simulink model "SHE_4_Angles"  (R2021a)
settings: Solver=daessc  StartTime=0.0  StopTime=.02*20  MaxStep=1e-6  RelTol=1e-3
libraries: spsIGBTDiodeLib x12, spsThreePhaseVIMeasurementLib x3, dsparch4 x2, spsDCVoltageSourceLib x2, spsRMSLib x2, simulink x2, spsVoltageMeasurementLib x2, spsAsynchronousMachineSIUnitsLib x1, spsGroundLib x1, spsThreePhaseSeriesRLCBranchLib x1, spspowerguiLib x1
settings Model: Creator=Ahmed Mohamed  LastModifiedBy=Ahmed Mohamed
settings SolverCC: ZeroCrossAlgorithm=Adaptive
settings DataIOCC: ReturnWorkspaceOutputs=off
settings DebuggingCC: IgnoredZcDiagnostic=none

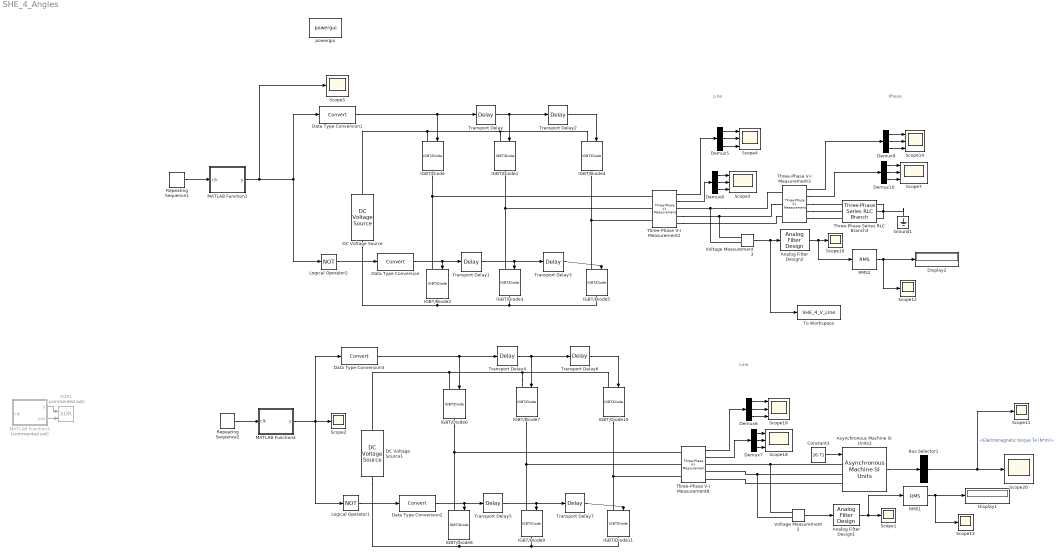
== system SHE_4_Angles ==
  note: Line
  note: Phase
  note: Line
  Analog Filter Design1 : dsparch4/Analog Filter Design  method=Butterworth  filttype=Lowpass  N=8  Wlo=2*pi*500  Whi=80  Rp=2  Rs=40
  Analog Filter Design2 : dsparch4/Analog Filter Design  method=Butterworth  filttype=Lowpass  N=8  Wlo=2*pi*550  Whi=80  Rp=2  Rs=40
  Asynchronous Machine SI Units2 : spsAsynchronousMachineSIUnitsLib/Asynchronous Machine SI Units  RotorType=Squirrel-cage  PresetModel="15:  5.4 HP (4KW)   400 V  50Hz 1430 RPM"  MechanicalLoad=Torque Tm  ShowDetailedParameters=on  ReferenceFrame=Rotor  Units=SI  MeasurementBus=off  NominalParameters=[4000 400 50]  VoltageRatio=1  Stator=[1.405 0.005839]  Rotor=[1.395 0.005839]  Cage1=[0.4155 0.002066]  Cage2=[0.4168 0.0003495]  Lm=0.1722  Mechanical=[0.0131 0.002985 2]  PolePairs=2  InitialConditions=[1 0 0 0 0 0 0 0]  SimulateSaturation=off  Saturation=[14.03593122, 27.81365428, 53.79336849, 72.68890987, 97.98006896, 148.6815601, 215.7428561, 302.9841135, 428.7778367 ; 230, 322, 414, 460, 506, 552, 598, 644, 690]  LoadFlowParameters=1492000  TsPowergui=0  TsBlock=-1  IterativeModel=Trapezoidal non iterative  IterativeDiscreteModel=Trapezoidal non iterative  Pmec=1.492e+006
  Bus Selector1 : BusSelector  OutputSignals=Mechanical.Electromagnetic torque Te (N*m)
  Constant3 : Constant  Value=26.71
  DC Voltage Source : spsDCVoltageSourceLib/DC Voltage Source  Amplitude=558.9759276  Measurements=None
  DC Voltage Source1 : spsDCVoltageSourceLib/DC Voltage Source  Amplitude=558.9759276  Measurements=None
  Data Type Conversion{,1..3} (4 alike) : DataTypeConversion
  Demux{5..10} (6 alike) : Demux  Outputs=3
  Display1 : Display
  Display2 : Display
  Ground1 : spsGroundLib/Ground  LConnTagsString=a
  IGBT/Diode{,1..11} (12 alike) : spsIGBTDiodeLib/IGBT//Diode  Ron=1e-3  Rs=1e5  Cs=inf  Measurements=off
  Logical Operator1 : Logic  Operator=NOT  AllPortsSameDT=off  OutDataTypeStr=boolean
  Logical Operator2 : Logic  Operator=NOT  AllPortsSameDT=off  OutDataTypeStr=boolean
  MATLAB Function1 : MATLAB Function  TreatAsAtomicUnit=on
  MATLAB Function3 : MATLAB Function  Commented=on  TreatAsAtomicUnit=on
  MATLAB Function4 : MATLAB Function  TreatAsAtomicUnit=on
  RMS1 : spsRMSLib/RMS  TrueRMS=off  Freq=50  RMSInit=0  Ts=0
  RMS2 : spsRMSLib/RMS  TrueRMS=off  Freq=50  RMSInit=0  Ts=0
  Repeating Sequence1 : simulink/Sources/Repeating Sequence  rep_seq_t=[0 .02]  rep_seq_y=[0 .02]
  Repeating Sequence2 : simulink/Sources/Repeating Sequence  rep_seq_t=[0 .02]  rep_seq_y=[0 .02]
  Scope{1..2,5,10..13,20} (8 alike) : Scope
  Scope{3..4,7,14,18..19} (6 alike) : Scope  NumInputPorts=3
  Three-Phase Series RLC Branch3 : spsThreePhaseSeriesRLCBranchLib/Three-Phase Series RLC Branch  LConnTagsString=A|B|C  RConnTagsString=A|B|C  BranchType=RL  Resistance=7.5*sqrt(2)  Inductance=7.5*sqrt(2)/314  Capacitance=1e-6  Measurements=None
  Three-Phase V-I Measurement2 : spsThreePhaseVIMeasurementLib/Three-Phase V-I Measurement  VoltageMeasurement=phase-to-phase  SetLabelV=off  LabelV=Vabc  Vpu=off  VpuLL=off  CurrentMeasurement=yes  SetLabelI=off  LabelI=Iabc  Ipu=off  Pbase=100e6  Vbase=500e3  OutputType=Complex  PhasorSimulation=off  PSBequivalent=0
  Three-Phase V-I Measurement3 : spsThreePhaseVIMeasurementLib/Three-Phase V-I Measurement  VoltageMeasurement=phase-to-ground  SetLabelV=off  LabelV=Vabc  Vpu=off  VpuLL=off  CurrentMeasurement=yes  SetLabelI=off  LabelI=Iabc  Ipu=off  Pbase=100e6  Vbase=500e3  OutputType=Complex  PhasorSimulation=off  PSBequivalent=0
  Three-Phase V-I Measurement8 : spsThreePhaseVIMeasurementLib/Three-Phase V-I Measurement  VoltageMeasurement=phase-to-phase  SetLabelV=off  LabelV=Vabc  Vpu=off  VpuLL=off  CurrentMeasurement=yes  SetLabelI=off  LabelI=Iabc  Ipu=off  Pbase=100e6  Vbase=500e3  OutputType=Complex  PhasorSimulation=off  PSBequivalent=0
  To Workspace : ToWorkspace  VariableName=SHE_4_V_Line  SaveFormat=Structure With Time  SampleTime=-1
  Transport Delay{,1..7} (8 alike) : TransportDelay  DelayTime=0.02/3  BufferSize=22480
  Voltage Measurement2 : spsVoltageMeasurementLib/Voltage Measurement  PhasorSimulation=off  OutputType=Complex  PSBequivalent=0
  Voltage Measurement3 : spsVoltageMeasurementLib/Voltage Measurement  PhasorSimulation=off  OutputType=Complex  PSBequivalent=0
  XOR1 : Logic  Commented=on  Operator=XOR  IconShape=distinctive  AllPortsSameDT=off  OutDataTypeStr=boolean
  powergui : spspowerguiLib/powergui  Priority=1  SimulationMode=Continuous  SampleTime=50e-6  frequency=60  Iterations=50  frequencyindice=0  Pbase=100e6  ErrMax=1e-4  UnitsV=kV  UnitsW=MW  buscounter=0  FunctionMessages=off  echomessages=off  EnableUseOfTLC=off  CurrentSourceSwitches=off  DisableSnubberDevices=off  DisableRonSwitches=off  DisableVfSwitches=off  DisplayEquations=off  AutomaticDiscreteSolvers=off  SolverType=Tustin/Backward Euler (TBE)  Interpol=off  ExternalGateDelay=off  methode=off  Ts=10  x0status=blocks  SPID=off  SwTol=0  HookPort=off  NonlinearTolerance=1e-4  nMaxIteration=100  ContinueOnMaxIteration=off  RestoreLinks=warning  ResistiveCurrentMeasurement=off  Frange=[0:2:500]  Ylog=off  Xlog=on  ShowGrid=off  save=off  variable=ZData  structure=Vout  ZoomFFT=off  StartTime=0.02  cycles=60  DisplayStyle=1  fundamental=50  FreqAxis=off  MaxFrequency=1000  frequencyindicesteady=1  RmsSteady=1  display=off
  wires:
  Transport Delay/1 -> Transport Delay2/1, IGBT/Diode1/1
  Transport Delay2/1 -> IGBT/Diode4/1
  Transport Delay3/1 -> IGBT/Diode5/1
  Data Type Conversion1/1 -> Transport Delay/1, IGBT/Diode/1
  Transport Delay1/1 -> Transport Delay3/1, IGBT/Diode3/1
  Data Type Conversion/1 -> Transport Delay1/1, IGBT/Diode2/1
  Logical Operator2/1 -> Data Type Conversion/1
  Repeating Sequence1/1 -> MATLAB Function1/1(clk)
  MATLAB Function1/1(y) -> Scope5/1, Data Type Conversion1/1, Logical Operator2/1
  MATLAB Function4/1(y) -> Scope2/1, Logical Operator1/1, Data Type Conversion3/1
  Repeating Sequence2/1 -> MATLAB Function4/1(clk)
  Logical Operator1/1 -> Data Type Conversion2/1
  Data Type Conversion2/1 -> IGBT/Diode8/1, Transport Delay5/1
  Transport Delay5/1 -> IGBT/Diode9/1, Transport Delay7/1
  Data Type Conversion3/1 -> Transport Delay4/1, IGBT/Diode6/1
  Transport Delay7/1 -> IGBT/Diode11/1
  Transport Delay6/1 -> IGBT/Diode10/1
  Transport Delay4/1 -> Transport Delay6/1, IGBT/Diode7/1
  RMS1/1 -> Scope13/1, Display1/1
  Demux6/3 -> Scope19/3
  Bus Selector1/1 -> Scope11/1, Scope20/1  "<Electromagnetic torque Te (N*m)>"
  Demux7/2 -> Scope18/2
  Asynchronous Machine SI Units2/1 -> Bus Selector1/1
  Demux7/1 -> Scope18/1
  Three-Phase V-I Measurement8/2 -> Demux7/1
  Three-Phase V-I Measurement8/1 -> Demux6/1
  Voltage Measurement2/1 -> Analog Filter Design1/1
  Constant3/1 -> Asynchronous Machine SI Units2/1
  Demux5/3 -> Scope4/3
  Demux9/1 -> Scope14/1
  Demux5/1 -> Scope4/1
  Demux10/3 -> Scope7/3
  Demux9/3 -> Scope14/3
  Analog Filter Design2/1 -> Scope10/1, RMS2/1
  Three-Phase V-I Measurement2/2 -> Demux8/1
  Demux5/2 -> Scope4/2
  Demux9/2 -> Scope14/2
  Demux8/2 -> Scope3/2
  Demux6/2 -> Scope19/2
  Demux7/3 -> Scope18/3
  Demux8/3 -> Scope3/3
  Demux10/2 -> Scope7/2
  Demux8/1 -> Scope3/1
  Three-Phase V-I Measurement2/1 -> Demux5/1
  Three-Phase V-I Measurement3/2 -> Demux10/1
  Analog Filter Design1/1 -> Scope1/1, RMS1/1
  Demux10/1 -> Scope7/1
  RMS2/1 -> Scope12/1, Display2/1
  Voltage Measurement3/1 -> To Workspace/1, Analog Filter Design2/1
  Three-Phase V-I Measurement3/1 -> Demux9/1
  Demux6/1 -> Scope19/1
  MATLAB Function3/1(y) -> XOR1/1
  MATLAB Function3/2(pos) -> XOR1/2
  connections:
  IGBT/Diode/RConn1 -- Three-Phase V-I Measurement2/LConn1 -- IGBT/Diode2/LConn1
  IGBT/Diode4/RConn1 -- Three-Phase V-I Measurement2/LConn3 -- IGBT/Diode5/LConn1
  IGBT/Diode2/RConn1 -- DC Voltage Source/LConn1 -- IGBT/Diode5/RConn1 -- IGBT/Diode3/RConn1
  IGBT/Diode1/LConn1 -- IGBT/Diode4/LConn1 -- DC Voltage Source/RConn1 -- IGBT/Diode/LConn1
  IGBT/Diode1/RConn1 -- Three-Phase V-I Measurement2/LConn2 -- IGBT/Diode3/LConn1
  IGBT/Diode6/RConn1 -- Three-Phase V-I Measurement8/LConn1 -- IGBT/Diode8/LConn1
  IGBT/Diode10/RConn1 -- IGBT/Diode11/LConn1 -- Three-Phase V-I Measurement8/LConn3
  IGBT/Diode8/RConn1 -- DC Voltage Source1/LConn1 -- IGBT/Diode9/RConn1 -- IGBT/Diode11/RConn1
  IGBT/Diode7/LConn1 -- DC Voltage Source1/RConn1 -- IGBT/Diode6/LConn1 -- IGBT/Diode10/LConn1
  IGBT/Diode7/RConn1 -- Three-Phase V-I Measurement8/LConn2 -- IGBT/Diode9/LConn1
  Three-Phase V-I Measurement8/RConn2 -- Asynchronous Machine SI Units2/LConn2 -- Voltage Measurement2/LConn2
  Three-Phase V-I Measurement2/RConn1 -- Three-Phase V-I Measurement3/LConn1 -- Voltage Measurement3/LConn2
  Three-Phase V-I Measurement3/LConn2 -- Three-Phase V-I Measurement2/RConn2 -- Voltage Measurement3/LConn1
  Three-Phase V-I Measurement8/RConn1 -- Asynchronous Machine SI Units2/LConn1 -- Voltage Measurement2/LConn1
  Ground1/LConn1 -- Three-Phase Series RLC Branch3/RConn2 -- Three-Phase Series RLC Branch3/RConn3 -- Three-Phase Series RLC Branch3/RConn1
  Three-Phase V-I Measurement3/RConn2 -- Three-Phase Series RLC Branch3/LConn2
  Asynchronous Machine SI Units2/LConn3 -- Three-Phase V-I Measurement8/RConn3
  Three-Phase V-I Measurement2/RConn3 -- Three-Phase V-I Measurement3/LConn3
  Three-Phase V-I Measurement3/RConn3 -- Three-Phase Series RLC Branch3/LConn3
  Three-Phase V-I Measurement3/RConn1 -- Three-Phase Series RLC Branch3/LConn1

== matlab function SHE_4_Angles/MATLAB Function3 ==
  data: clk input; y output; pos output
function [y, pos]   = fcn(clk)
alpha_1 = 9.836918511590010;
alpha_2 = 15.075614954744452;
alpha_3 = 85.053395836851310;
alpha_4 = 86.272553966387690;

% alpha_1 = 10.545613174205297;
% alpha_2 = 16.092458911934940;
% alpha_3 = 30.904552394074074;
% alpha_4 = 32.866886824016426;

ts1 = (alpha_1/360) * .02; % 1.11111 mS
ts2 = (alpha_2/360) * .02; % 2.22222 mS
ts3 = (alpha_3/360) * .02; % 3.33333 mS
ts4 = (alpha_4/360) * .02; % 4.44444 mS
ts6 = .01 - ts4;
ts7 = .01 - ts3;
ts8 = .01 - ts2;
ts9 = .01 - ts1;
ts10 = .01;

if clk>.01
    clk = clk - .01;
    pos = 1;
else
    pos = 0;
end

if clk <= ts1
    y = 1;
elseif clk <= ts2
    y = 0;
elseif clk <= ts3
    y = 1;
elseif clk <= ts4
    y = 0;
elseif clk <= ts6
    y = 1;
elseif clk <= ts7
    y = 0;
elseif clk <= ts8
    y = 1;
elseif clk <= ts9
    y = 0;
elseif clk <= ts10
    y = 1;
else
    y = 0;
end

== matlab function SHE_4_Angles/MATLAB Function4 ==
  data: clk input; y output
function y    = get_SHE4_Pulses(clk)
alpha_1 = 9.836918511590010;
alpha_2 = 15.075614954744452;
alpha_3 = 85.053395836851310;
alpha_4 = 86.272553966387690;

ts1 = (alpha_1/360) * .02;
ts2 = (alpha_2/360) * .02;
ts3 = (alpha_3/360) * .02;
ts4 = (alpha_4/360) * .02;
ts6 = .01 - ts4;
ts7 = .01 - ts3;
ts8 = .01 - ts2;
ts9 = .01 - ts1;
ts10 = .01;

if clk>.01
    clk = clk - .01;
    pos = 1;
else
    pos = 0;
end

if clk <= ts1
    y = xor(1, pos);
elseif clk <= ts2
    y = xor(0, pos);
elseif clk <= ts3
    y = xor(1, pos);
elseif clk <= ts4
    y = xor(0, pos);
elseif clk <= ts6
    y = xor(1, pos);
elseif clk <= ts7
    y = xor(0, pos);
elseif clk <= ts8
    y = xor(1, pos);
elseif clk <= ts9
    y = xor(0, pos);
elseif clk <= ts10
    y = xor(1, pos);
else
    y = xor(0, pos);
end

== matlab function SHE_4_Angles/MATLAB Function1 ==
  data: clk input; y output
function y    = get_SHE4_Pulses(clk)
alpha_1 = 9.836918511590010;
alpha_2 = 15.075614954744452;
alpha_3 = 85.053395836851310;
alpha_4 = 86.272553966387690;

ts1 = (alpha_1/360) * .02;
ts2 = (alpha_2/360) * .02;
ts3 = (alpha_3/360) * .02;
ts4 = (alpha_4/360) * .02;
ts6 = .01 - ts4;
ts7 = .01 - ts3;
ts8 = .01 - ts2;
ts9 = .01 - ts1;
ts10 = .01;

if clk>.01
    clk = clk - .01;
    pos = 1;
else
    pos = 0;
end

if clk <= ts1
    y = xor(1, pos);
elseif clk <= ts2
    y = xor(0, pos);
elseif clk <= ts3
    y = xor(1, pos);
elseif clk <= ts4
    y = xor(0, pos);
elseif clk <= ts6
    y = xor(1, pos);
elseif clk <= ts7
    y = xor(0, pos);
elseif clk <= ts8
    y = xor(1, pos);
elseif clk <= ts9
    y = xor(0, pos);
elseif clk <= ts10
    y = xor(1, pos);
else
    y = xor(0, pos);
end
